simulink model "Sequ_exam"  (R2025b)
settings: Solver=VariableStepAuto  StartTime=0.0  StopTime=9.5  FixedStep=0.01  RelTol=1e-3
libraries: simulink_extras x1, SignalEditorBlockLib x1
settings Model: PacingRate=1.100000  Creator=Soochan Kim  LastModifiedBy=Soochan Kim

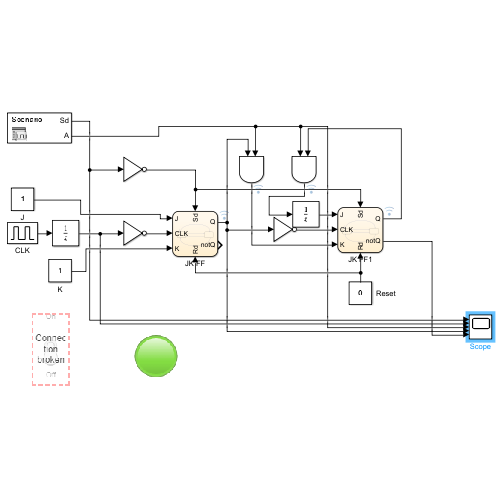
[thumbnail: Simulink's stored preview of the top-level diagram]
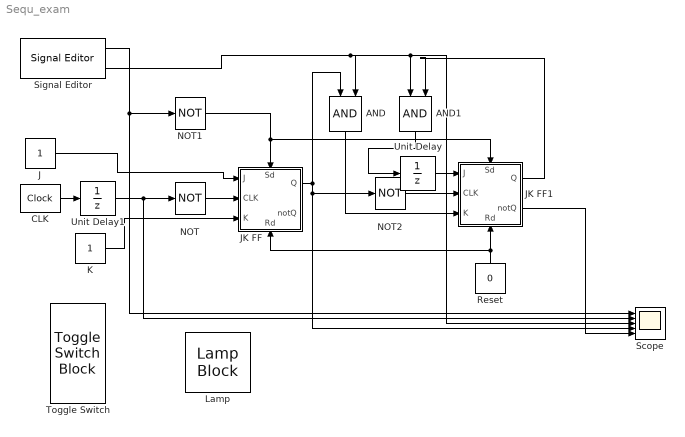
== system Sequ_exam ==
  AND : Logic  IconShape=distinctive  AllPortsSameDT=off  OutDataTypeStr=boolean
  AND1 : Logic  IconShape=distinctive  AllPortsSameDT=off  OutDataTypeStr=boolean
  CLK : simulink_extras/Flip Flops/Clock  period=1
  J : Constant
  JK FF : Stateflow chart  TreatAsAtomicUnit=on
      settings: PortSchema="{\"entries\":[{\"content\":{\"sides\":[{\"content\":{\"connectorIds\":[\"In1\",\"In2\",\"In3\"]},\"type\":\"ConnectorPlacement.EquallySpacedRectSide\",\"uuid\":\"2af75eb2-b907-44b2-82cc-b57e0a0d1c9b\"},{\"content\":{\"connectorIds\":[\"Out1\",\"Out2\"],\"side\":\"RIGHT\"},\"type\":\"ConnectorPlacement.EquallySpacedRectSide\",\"uuid\":\"6517b60d-825e-4e21-aa23-d5468b780dc3\"},{\"content\":{\"connectorIds\":[\"In4\"],\"side\":\"TOP\"},\"type\":\"ConnectorPlacement.EquallySpacedRectSide\",\"uuid\":\"6792e8eb-5222-4842-ba8a-bb88748afe2e\"},{\"content\":{\"connectorIds\":[\"In5\"],\"side\":\"BOTTOM\"},\"type\":\"ConnectorPlacement.EquallySpacedRectSide\",\"uuid\":\"cabb32ad-94a1-4a96-98a9-7356dbac5a93\"}]},\"type\":\"ConnectorPlacement.EquallySpacedConnector\",\"uuid\":\"0f8d812c-ded7-4acb-bdb8-74f44742dfe2\"}],\"packageUris\":[\"http://schema.mathworks.com/mf0/Connector/R2020b\"],\"version\":\"1.0\"}"
  JK FF1 : Stateflow chart  TreatAsAtomicUnit=on
      settings: PortSchema="{\"entries\":[{\"content\":{\"sides\":[{\"content\":{\"connectorIds\":[\"In1\",\"In2\",\"In3\"]},\"type\":\"ConnectorPlacement.EquallySpacedRectSide\",\"uuid\":\"2af75eb2-b907-44b2-82cc-b57e0a0d1c9b\"},{\"content\":{\"connectorIds\":[\"Out1\",\"Out2\"],\"side\":\"RIGHT\"},\"type\":\"ConnectorPlacement.EquallySpacedRectSide\",\"uuid\":\"6517b60d-825e-4e21-aa23-d5468b780dc3\"},{\"content\":{\"connectorIds\":[\"In4\"],\"side\":\"TOP\"},\"type\":\"ConnectorPlacement.EquallySpacedRectSide\",\"uuid\":\"6792e8eb-5222-4842-ba8a-bb88748afe2e\"},{\"content\":{\"connectorIds\":[\"In5\"],\"side\":\"BOTTOM\"},\"type\":\"ConnectorPlacement.EquallySpacedRectSide\",\"uuid\":\"cabb32ad-94a1-4a96-98a9-7356dbac5a93\"}]},\"type\":\"ConnectorPlacement.EquallySpacedConnector\",\"uuid\":\"0f8d812c-ded7-4acb-bdb8-74f44742dfe2\"}],\"packageUris\":[\"http://schema.mathworks.com/mf0/Connector/R2020b\"],\"version\":\"1.0\"}"
  K : Constant
  Lamp : LampBlock  LabelPosition=Hide  DefaultColor=[192.0, 192.0, 192.0]
  NOT : Logic  Operator=NOT  IconShape=distinctive  AllPortsSameDT=off  OutDataTypeStr=boolean
  NOT1 : Logic  Operator=NOT  IconShape=distinctive  AllPortsSameDT=off  OutDataTypeStr=boolean
  NOT2 : Logic  Operator=NOT  IconShape=distinctive  AllPortsSameDT=off  OutDataTypeStr=boolean
  Reset : Constant  Value=0
  Scope : Scope  NumInputPorts=5
      settings: ActiveDisplayYMinimum=-0.12499999999999997  ActiveDisplayYMaximum=1.125
  Signal Editor : SignalEditorBlockLib/Signal Editor  FileName=sig_A.mat  ActiveScenario=Scenario  ActiveSignal=Sd  IsBus=off  OutputBusObjectStr=Bus: BusObject  SampleTime=0  ZeroCross=off  OutputAfterFinalValue=Setting to zero  Unit=inherit  PreserveSignalName=on  ApplySigPropsToAllScenarios=on  ApplySigPropsToAllSignals=off  SignalPropertySource=Dialog parameters
  Toggle Switch : ToggleSwitchBlock
  Unit Delay : UnitDelay  SampleTime=0.01  HasFrameUpgradeWarning=on
  Unit Delay1 : UnitDelay  SampleTime=0.5  HasFrameUpgradeWarning=on
  wires:
  J/1 -> JK FF/1(J)
  K/1 -> JK FF/3(K)
  CLK/1 -> Unit Delay1/1
  Reset/1 -> JK FF/5(Rd), JK FF1/5(Rd)
  NOT/1 -> JK FF/2(CLK)
  NOT1/1 -> JK FF1/4(Sd), JK FF/4(Sd)
  AND/1 -> JK FF1/3(K)
  NOT2/1 -> JK FF1/2(CLK)
  JK FF1/1(Q) -> AND1/2
  Unit Delay1/1 -> Scope/2, NOT/1
  JK FF/1(Q) -> Scope/4, NOT2/1, AND/1
  Signal Editor/1 -> Scope/1, NOT1/1
  Signal Editor/2 -> Scope/3, AND1/1, AND/2
  JK FF1/2(notQ) -> Scope/5
  Unit Delay/1 -> JK FF1/1(J)
  AND1/1 -> Unit Delay/1

== stateflow chart Sequ_exam/JK FF1 ==
  settings: updateMethod=DISCRETE  sampleTime=0.01
  state State_Q0
    entry:
    Q=0;
    notQ=1;
  state State_Q1
    entry:
    Q=1;
    notQ=0;
  State_Q0 -> State_Q1 [order 1] : [Sd==1 && Rd==0]
  (default) -> State_Q0
  State_Q0 -> State_Q1 [order 2] : [Rd == 0 && Sd == 0 && rising(CLK) && J==1]
  State_Q1 -> State_Q0 [order 2] : [Rd == 0 && Sd == 0 && rising(CLK) && K==1]
  State_Q1 -> State_Q0 [order 1] : [Rd==1]
  data: J input; Q output; CLK input; K input; Sd input; Rd input; notQ output

== stateflow chart Sequ_exam/JK FF ==
  settings: updateMethod=DISCRETE  sampleTime=0.01
  state State_Q0
    entry:
    Q=0;
    notQ=1;
  state State_Q1
    entry:
    Q=1;
    notQ=0;
  State_Q0 -> State_Q1 [order 1] : [Sd==1 && Rd==0]
  (default) -> State_Q0
  State_Q0 -> State_Q1 [order 2] : [Rd == 0 && Sd == 0 && rising(CLK) && J==1]
  State_Q1 -> State_Q0 [order 2] : [Rd == 0 && Sd == 0 && rising(CLK) && K==1]
  State_Q1 -> State_Q0 [order 1] : [Rd==1]
  data: J input; Q output; CLK input; K input; Sd input; Rd input; notQ output
